simulink model "DynJointVerify"  (Simulink 7.6)
settings: Solver=ode45  StartTime=0.0  StopTime=8  RelTol=1e-3
InitFcn:
  | eval('Config.m')
values from neighbouring files (symbols this model uses):
  a2 = 0    [Config.m]    (also in CtrPlatformCfg.m)
  a3 = 0    [Config.m]    (also in CtrPlatformCfg.m)
  a4 = 0    [Config.m]    (also in CtrPlatformCfg.m)
  a5 = 90    [Config.m]    (also in CtrPlatformCfg.m)
  a6 = 0    [Config.m]    (also in CtrPlatformCfg.m)
  Cen = Cen(:)'    [Config.m]    (also in CtrPlatformCfg.m; DynEulerTest.m = Cen'; EfDynCAD.m = [cen1,cen2,cen3,cen4,cen5,cen6]')
  freq = tvel/radius    (= 1)    [Config.m]    (also in CtrPlatformCfg.m)
  Gravity = 9.8    [Config.m]    (also in CtrPlatformCfg.m)
  Ie1 = in1(:)'    [Config.m]    (also in CtrPlatformCfg.m; DynEulerTest.m = in1(:); EfDynCAD.m = in1(:))
  Ie2 = in2(:)'    [Config.m]    (also in CtrPlatformCfg.m; DynEulerTest.m = in2(:); EfDynCAD.m = in2(:))
  Ie3 = in3(:)'    [Config.m]    (also in CtrPlatformCfg.m; DynEulerTest.m = in3(:); EfDynCAD.m = in3(:))
  Ie4 = in4(:)'    [Config.m]    (also in CtrPlatformCfg.m; DynEulerTest.m = in4(:); EfDynCAD.m = in4(:))
  Ie5 = in5(:)'    [Config.m]    (also in CtrPlatformCfg.m; DynEulerTest.m = in5(:); EfDynCAD.m = in5(:))
  Ie6 = in6(:)'    [Config.m]    (also in CtrPlatformCfg.m; DynEulerTest.m = in6(:); EfDynCAD.m = in6(:))
  in1 = [5.2954 -0.2565 -0.6366;-0.2565 4.7000 0.2830;-0.6366 0.2829 5.8635]    [Config.m]    (also in CtrPlatformCfg.m; DynEulerTest.m; EfDynCAD.m = [0.54  -0.01 0.23)
  in2 = [5.8840 0.0072 0.0135;0.0072 6.0178 -0.1907;0.0135 -0.1907 0.3374]    [Config.m]    (also in CtrPlatformCfg.m; DynEulerTest.m; EfDynCAD.m = (R_x*R_z)*in2*(R_x*R_z)')
  in3 = [1.8201 -0.2274 -0.3112;-0.2274 2.2537 -0.1441;-0.3112 -0.1441 1.9485]    [Config.m]    (also in CtrPlatformCfg.m; DynEulerTest.m; EfDynCAD.m = (R_x*R_z)*in3*(R_x*R_z)')
  in4 = [0.0607 -0.0922 0;-0.0922 1.4493 0;0 0 1.4620]    [Config.m]    (also in CtrPlatformCfg.m; DynEulerTest.m = [0.0607 -0.0922 0;-0.0922 1.4493 0;0 0,1.4620]; EfDynCAD.m = (R_y*Rz)*in4*(R_y*Rz)')
  in5 = [0.0191 0.0032 0;0.0032 0.0228 0;0 0 0.0291]    [Config.m]    (also in CtrPlatformCfg.m; DynEulerTest.m; EfDynCAD.m = (R_x*R_y)*in5*(R_x*R_y)')
  in6 = [0.0012 0 0;0 0.0007 0;0 0 0.0007]    [Config.m]    (also in CtrPlatformCfg.m; DynEulerTest.m; EfDynCAD.m = (R_y*Rz)*in6*(R_y*Rz)')
  init_Endx = gd_init(1,4)    [Config.m]    (also in CtrPlatformCfg.m)
  init_Endy = gd_init(2,4)    [Config.m]    (also in CtrPlatformCfg.m)
  init_Endz = gd_init(3,4)    [Config.m]    (also in CtrPlatformCfg.m)
  init_Rot = gd_init(1:3,1:3)    [Config.m]    (also in CtrPlatformCfg.m)
  L = [l1 l2 l3 l4 l5 l6 l7 l8 l9]    [Config.m]    (also in CtrPlatformCfg.m)
  Ma = [ma1 ma2 ma3 ma4 ma5 ma6]    [Config.m]    (also in CtrPlatformCfg.m; DynEulerTest.m = [ma1; ma2; ma3; ma4; ma5; ma6]; EfDynCAD.m = [ma1 ma2 ma3 ma4 ma5 ma6]')
  tvel = 120    [Config.m]    (also in CtrPlatformCfg.m)
undefined symbols (not defined in the file or in its folder): a1, L_EU
libraries: mblibv1 x41, simulink x7
(part 2 of 2)

== system DynJointVerify/Dynamic/Largrange ==
  In1 : Inport
  BodyVel : Stateflow chart  TreatAsAtomicUnit=on
  C*Omega : Stateflow chart  TreatAsAtomicUnit=on
  Demux : Demux  Outputs=3
  M*Acc : Stateflow chart  TreatAsAtomicUnit=on
  N : Stateflow chart  TreatAsAtomicUnit=on
  Sum : Sum  Inputs=+++
  Force : Outport
  Acc : Outport  Port=2
  Potential : Outport  Port=3
  Cori : Outport  Port=4
  LaVel : Outport  Port=5
  wires:
  M*Acc/1(M_Acc) -> Sum/1, Acc/1
  C*Omega/1(C_Omega) -> Sum/3, Cori/1
  Demux/1 -> M*Acc/2(EnTheta), N/1(EnTheta), C*Omega/2(EnTheta), BodyVel/1(EnTheta)
  Demux/2 -> C*Omega/1(RefOmega), C*Omega/3(EnOmega), BodyVel/2(EnOmega)
  Demux/3 -> M*Acc/1(RefAcc)
  N/1(N) -> Sum/2, Potential/1
  In1/1 -> Demux/1
  Sum/1 -> Force/1
  BodyVel/1(Vel) -> LaVel/1

== system DynJointVerify/Dynamic/Potential Force ==
  In1 : Inport
  In2 : Inport  Port=2
  Demux : Demux  Outputs=6
  Demux1 : Demux  Outputs=6
  Err{1..6} (6 alike) : Scope
      Err1 settings: SaveName=ScopeData6
      Err2 settings: SaveName=ScopeData7
      Err3 settings: TimeRange=3  YMin=-6e-014  YMax=6e-014  SaveName=ScopeData8
      Err4 settings: SaveName=ScopeData9
      Err5 settings: SaveName=ScopeData10
      Err6 settings: SaveName=ScopeData11
  R1 Force : Scope  NumInputPorts=2
      settings: TimeRange=10  YMin=-2.999999999999999e-017~-1  YMax=4e-017~1
  R2 Force : Scope  NumInputPorts=2
      settings: YMin=-5~-5  YMax=5~5
  R3 Force : Scope  NumInputPorts=2
      settings: TimeRange=3  YMin=-227.5~-226.42678523  YMax=-225~-226.42678517  SaveName=ScopeData2
  R4 Force : Scope  NumInputPorts=2
      settings: YMin=-5~-5  YMax=5~5  SaveName=ScopeData3
  R5 Force : Scope  NumInputPorts=2
      settings: YMin=-5~-5  YMax=5~5  SaveName=ScopeData4
  R6 Force : Scope  NumInputPorts=2
      settings: YMin=-5~-5  YMax=5~5  SaveName=ScopeData5
  Sum{,1..5} (6 alike) : Sum  Inputs=+|-
  wires:
  In2/1 -> Demux1/1
  In1/1 -> Demux/1
  Sum/1 -> Err1/1
  Sum1/1 -> Err2/1
  Sum2/1 -> Err3/1
  Sum3/1 -> Err4/1
  Sum4/1 -> Err5/1
  Sum5/1 -> Err6/1
  Demux/1 -> Sum/1, R1 Force/1
  Demux1/1 -> Sum/2, R1 Force/2
  Demux/2 -> R2 Force/1, Sum1/1
  Demux/3 -> R3 Force/1, Sum2/1
  Demux/4 -> R4 Force/1, Sum3/1
  Demux/5 -> R5 Force/1, Sum4/1
  Demux/6 -> R6 Force/1, Sum5/1
  Demux1/2 -> R2 Force/2, Sum1/2
  Demux1/3 -> R3 Force/2, Sum2/2
  Demux1/4 -> R4 Force/2, Sum3/2
  Demux1/5 -> R5 Force/2, Sum4/2
  Demux1/6 -> R6 Force/2, Sum5/2

== system DynJointVerify/Error Analysis/Euler ==
  In1 : Inport
  In2 : Inport  Port=2
  Demux : Demux  Outputs=6
  Demux1 : Demux  Outputs=6
  Err{1..6} (6 alike) : Scope
      Err1 settings: SaveName=ScopeData6
      Err2 settings: SaveName=ScopeData7
      Err3 settings: TimeRange=3  YMin=-6e-014  YMax=6e-014  SaveName=ScopeData8
      Err4 settings: SaveName=ScopeData9
      Err5 settings: SaveName=ScopeData10
      Err6 settings: SaveName=ScopeData11
  R1 Force : Scope  NumInputPorts=2
      settings: TimeRange=10  YMin=-2.999999999999999e-017~-1  YMax=4e-017~1
  R2 Force : Scope  NumInputPorts=2
      settings: YMin=-5~-5  YMax=5~5
  R3 Force : Scope  NumInputPorts=2
      settings: TimeRange=3  YMin=-227.5~-226.42678523  YMax=-225~-226.42678517  SaveName=ScopeData2
  R4 Force : Scope  NumInputPorts=2
      settings: YMin=-5~-5  YMax=5~5  SaveName=ScopeData3
  R5 Force : Scope  NumInputPorts=2
      settings: YMin=-5~-5  YMax=5~5  SaveName=ScopeData4
  R6 Force : Scope  NumInputPorts=2
      settings: YMin=-5~-5  YMax=5~5  SaveName=ScopeData5
  Sum{,1..5} (6 alike) : Sum  Inputs=+|-
  wires:
  In2/1 -> Demux1/1
  In1/1 -> Demux/1
  Sum/1 -> Err1/1
  Sum1/1 -> Err2/1
  Sum2/1 -> Err3/1
  Sum3/1 -> Err4/1
  Sum4/1 -> Err5/1
  Sum5/1 -> Err6/1
  Demux/1 -> R1 Force/1, Sum/1
  Demux1/1 -> R1 Force/2, Sum/2
  Demux/2 -> Sum1/1, R2 Force/1
  Demux/3 -> Sum2/1, R3 Force/1
  Demux/4 -> Sum3/1, R4 Force/1
  Demux/5 -> Sum4/1, R5 Force/1
  Demux/6 -> Sum5/1, R6 Force/1
  Demux1/2 -> Sum1/2, R2 Force/2
  Demux1/3 -> Sum2/2, R3 Force/2
  Demux1/4 -> Sum3/2, R4 Force/2
  Demux1/5 -> Sum4/2, R5 Force/2
  Demux1/6 -> Sum5/2, R6 Force/2

== system DynJointVerify/Error Analysis/Largrange ==
  In1 : Inport
  In2 : Inport  Port=2
  Demux : Demux  Outputs=6
  Demux1 : Demux  Outputs=6
  Err{1..6} (6 alike) : Scope
      Err1 settings: SaveName=ScopeData6
      Err2 settings: SaveName=ScopeData7
      Err3 settings: TimeRange=3  YMin=-6e-014  YMax=6e-014  SaveName=ScopeData8
      Err4 settings: SaveName=ScopeData9
      Err5 settings: SaveName=ScopeData10
      Err6 settings: SaveName=ScopeData11
  R1 Force : Scope  NumInputPorts=2
      settings: TimeRange=10  YMin=-2.999999999999999e-017~-1  YMax=4e-017~1
  R2 Force : Scope  NumInputPorts=2
      settings: YMin=-5~-5  YMax=5~5
  R3 Force : Scope  NumInputPorts=2
      settings: TimeRange=3  YMin=-227.5~-226.42678523  YMax=-225~-226.42678517  SaveName=ScopeData2
  R4 Force : Scope  NumInputPorts=2
      settings: YMin=-5~-5  YMax=5~5  SaveName=ScopeData3
  R5 Force : Scope  NumInputPorts=2
      settings: YMin=-5~-5  YMax=5~5  SaveName=ScopeData4
  R6 Force : Scope  NumInputPorts=2
      settings: YMin=-5~-5  YMax=5~5  SaveName=ScopeData5
  Sum{,1..5} (6 alike) : Sum  Inputs=+|-
  wires:
  Sum/1 -> Err1/1
  Sum1/1 -> Err2/1
  Sum2/1 -> Err3/1
  Sum3/1 -> Err4/1
  Sum4/1 -> Err5/1
  Sum5/1 -> Err6/1
  Demux/1 -> Sum/1, R1 Force/1
  Demux1/1 -> Sum/2, R1 Force/2
  Demux/2 -> R2 Force/1, Sum1/1
  Demux/3 -> R3 Force/1, Sum2/1
  Demux/4 -> R4 Force/1, Sum3/1
  Demux/5 -> R5 Force/1, Sum4/1
  Demux/6 -> R6 Force/1, Sum5/1
  Demux1/2 -> R2 Force/2, Sum1/2
  Demux1/3 -> R3 Force/2, Sum2/2
  Demux1/4 -> R4 Force/2, Sum3/2
  Demux1/5 -> R5 Force/2, Sum4/2
  Demux1/6 -> R6 Force/2, Sum5/2
  In1/1 -> Demux/1
  In2/1 -> Demux1/1

== system DynJointVerify/Error Analysis/VelDisplay ==
  In1 : Inport
  In4 : Inport  Port=2
  Demux3 : Demux  Outputs=6
  Demux4 : Demux  Outputs=6
  Jnt1 : Subsystem
  Jnt2 : Subsystem
  Jnt3 : Subsystem
  Jnt4 : Subsystem
  Jnt5 : Subsystem
  Jnt6 : Subsystem
  wires:
  In1/1 -> Demux4/1
  In4/1 -> Demux3/1
  Demux4/1 -> Jnt1/1(In1)
  Demux3/1 -> Jnt1/2(In2)
  Demux4/2 -> Jnt2/1(In1)
  Demux3/2 -> Jnt2/2(In2)
  Demux4/3 -> Jnt3/1(In1)
  Demux3/3 -> Jnt3/2(In2)
  Demux4/4 -> Jnt4/1(In1)
  Demux3/4 -> Jnt4/2(In2)
  Demux4/5 -> Jnt5/1(In1)
  Demux3/5 -> Jnt5/2(In2)
  Demux4/6 -> Jnt6/1(In1)
  Demux3/6 -> Jnt6/2(In2)

== system DynJointVerify/Fanuc/ BodySensor 1 ==
  Avx : Scope
      settings: TimeRange=3  YMin=-150  YMax=125  SaveName=ScopeData62
  Avy : Scope
      settings: TimeRange=3  YMin=-150  YMax=125  SaveName=ScopeData63
  Avz : Scope
      settings: TimeRange=3  YMin=-150  YMax=125  SaveName=ScopeData64
  Awx : Scope
      settings: TimeRange=3  YMin=-150  YMax=125  SaveName=ScopeData65
  Awy : Scope
      settings: TimeRange=3  YMin=-150  YMax=125  SaveName=ScopeData66
  Awz : Scope
      settings: TimeRange=3  YMin=-150  YMax=125  SaveName=ScopeData67
  "Body Sensor " : mblibv1/Sensors &  Actuators/Body Sensor  DialogController=MECH.DynMechDlgSource  SystemSampleTime=-1  UpdateFromCAD=off  PhysicalDomain=Mechanical  PortType=blob  Muxed=on  Pose=off  Angle=on  AngleUnits=deg  ArcVelocity=on  ArcVelocityUnits=deg/s  ArcAcceleration=on  ArcAccelerationUnits=deg/s^2  CoordPosition=off  CoordPositionUnits=mm  Velocity=on  VelocityUnits=mm/s  Acceleration=on  AccelerationUnits=mm/s^2  Quaternion=on  QuaternionDT=off  QuaternionDDT=off  QuaternionUnits=off  OutputVector=[1]  ActiveIO=on  Width=12  DialogClass=MechanicalSensorBlock  ReferenceFrame=Local (Body CS)
  Demux5 : Demux  Outputs=12
  Vx : Scope
      settings: TimeRange=3  YMin=-150  YMax=125  SaveName=ScopeData55
  Vy : Scope
      settings: TimeRange=3  YMin=-150  YMax=125  SaveName=ScopeData57
  Vz : Scope
      settings: TimeRange=3  YMin=-150  YMax=125  SaveName=ScopeData58
  wx : Scope
      settings: TimeRange=3  YMin=-150  YMax=125  SaveName=ScopeData59
  wy : Scope
      settings: TimeRange=3  YMin=-150  YMax=125  SaveName=ScopeData60
  wz : Scope
      settings: TimeRange=3  YMin=-150  YMax=125  SaveName=ScopeData61
  Conn1 : PMIOPort  Port=1  Side=Left
  Out : Outport
  wires:
  "Body Sensor "/1 -> Out/1, Demux5/1
  Demux5/1 -> Vx/1
  Demux5/2 -> Vy/1
  Demux5/3 -> Vz/1
  Demux5/4 -> wx/1
  Demux5/5 -> wy/1
  Demux5/6 -> wz/1
  Demux5/7 -> Avx/1
  Demux5/8 -> Avy/1
  Demux5/9 -> Avz/1
  Demux5/10 -> Awx/1
  Demux5/11 -> Awy/1
  Demux5/12 -> Awz/1
  connections:
  Conn1/RConn1 -- "Body Sensor "/LConn1

== system DynJointVerify/Fanuc/ BodySensor 2 ==
  Avx : Scope
      settings: TimeRange=3  YMin=-150  YMax=125  SaveName=ScopeData62
  Avy : Scope
      settings: TimeRange=3  YMin=-150  YMax=125  SaveName=ScopeData63
  Avz : Scope
      settings: TimeRange=3  YMin=-150  YMax=125  SaveName=ScopeData64
  Awx : Scope
      settings: TimeRange=3  YMin=-150  YMax=125  SaveName=ScopeData65
  Awy : Scope
      settings: TimeRange=3  YMin=-150  YMax=125  SaveName=ScopeData66
  Awz : Scope
      settings: TimeRange=3  YMin=-150  YMax=125  SaveName=ScopeData67
  "Body Sensor " : mblibv1/Sensors &  Actuators/Body Sensor  DialogController=MECH.DynMechDlgSource  SystemSampleTime=-1  UpdateFromCAD=off  PhysicalDomain=Mechanical  PortType=blob  Muxed=on  Pose=off  Angle=on  AngleUnits=deg  ArcVelocity=on  ArcVelocityUnits=deg/s  ArcAcceleration=on  ArcAccelerationUnits=deg/s^2  CoordPosition=off  CoordPositionUnits=mm  Velocity=on  VelocityUnits=mm/s  Acceleration=on  AccelerationUnits=mm/s^2  Quaternion=on  QuaternionDT=off  QuaternionDDT=off  QuaternionUnits=off  OutputVector=[1]  ActiveIO=on  Width=12  DialogClass=MechanicalSensorBlock  ReferenceFrame=Local (Body CS)
  Demux5 : Demux  Outputs=12
  Vx : Scope
      settings: TimeRange=3  YMin=-150  YMax=125  SaveName=ScopeData55
  Vy : Scope
      settings: TimeRange=3  YMin=-150  YMax=125  SaveName=ScopeData57
  Vz : Scope
      settings: TimeRange=3  YMin=-150  YMax=125  SaveName=ScopeData58
  wx : Scope
      settings: TimeRange=3  YMin=-150  YMax=125  SaveName=ScopeData59
  wy : Scope
      settings: TimeRange=3  YMin=-150  YMax=125  SaveName=ScopeData60
  wz : Scope
      settings: TimeRange=3  YMin=-150  YMax=125  SaveName=ScopeData61
  Conn1 : PMIOPort  Port=1  Side=Left
  Out : Outport
  wires:
  Demux5/12 -> Awz/1
  Demux5/11 -> Awy/1
  Demux5/10 -> Awx/1
  Demux5/9 -> Avz/1
  Demux5/8 -> Avy/1
  Demux5/7 -> Avx/1
  Demux5/6 -> wz/1
  Demux5/5 -> wy/1
  Demux5/4 -> wx/1
  Demux5/3 -> Vz/1
  Demux5/2 -> Vy/1
  Demux5/1 -> Vx/1
  "Body Sensor "/1 -> Demux5/1, Out/1
  connections:
  Conn1/RConn1 -- "Body Sensor "/LConn1

== system DynJointVerify/Fanuc/ BodySensor 3 ==
  Avx : Scope
      settings: TimeRange=3  YMin=-150  YMax=125  SaveName=ScopeData62
  Avy : Scope
      settings: TimeRange=3  YMin=-150  YMax=125  SaveName=ScopeData63
  Avz : Scope
      settings: TimeRange=3  YMin=-150  YMax=125  SaveName=ScopeData64
  Awx : Scope
      settings: TimeRange=3  YMin=-150  YMax=125  SaveName=ScopeData65
  Awy : Scope
      settings: TimeRange=3  YMin=-150  YMax=125  SaveName=ScopeData66
  Awz : Scope
      settings: TimeRange=3  YMin=-150  YMax=125  SaveName=ScopeData67
  "Body Sensor " : mblibv1/Sensors &  Actuators/Body Sensor  DialogController=MECH.DynMechDlgSource  SystemSampleTime=-1  UpdateFromCAD=off  PhysicalDomain=Mechanical  PortType=blob  Muxed=on  Pose=off  Angle=on  AngleUnits=deg  ArcVelocity=on  ArcVelocityUnits=deg/s  ArcAcceleration=on  ArcAccelerationUnits=deg/s^2  CoordPosition=off  CoordPositionUnits=mm  Velocity=on  VelocityUnits=mm/s  Acceleration=on  AccelerationUnits=mm/s^2  Quaternion=on  QuaternionDT=off  QuaternionDDT=off  QuaternionUnits=off  OutputVector=[1]  ActiveIO=on  Width=12  DialogClass=MechanicalSensorBlock  ReferenceFrame=Local (Body CS)
  Demux5 : Demux  Outputs=12
  Vx : Scope
      settings: TimeRange=3  YMin=-150  YMax=125  SaveName=ScopeData55
  Vy : Scope
      settings: TimeRange=3  YMin=-150  YMax=125  SaveName=ScopeData57
  Vz : Scope
      settings: TimeRange=3  YMin=-150  YMax=125  SaveName=ScopeData58
  wx : Scope
      settings: TimeRange=3  YMin=-150  YMax=125  SaveName=ScopeData59
  wy : Scope
      settings: TimeRange=3  YMin=-150  YMax=125  SaveName=ScopeData60
  wz : Scope
      settings: TimeRange=3  YMin=-150  YMax=125  SaveName=ScopeData61
  Conn1 : PMIOPort  Port=1  Side=Left
  Out : Outport
  wires:
  "Body Sensor "/1 -> Out/1, Demux5/1
  Demux5/1 -> Vx/1
  Demux5/2 -> Vy/1
  Demux5/3 -> Vz/1
  Demux5/4 -> wx/1
  Demux5/5 -> wy/1
  Demux5/6 -> wz/1
  Demux5/7 -> Avx/1
  Demux5/8 -> Avy/1
  Demux5/9 -> Avz/1
  Demux5/10 -> Awx/1
  Demux5/11 -> Awy/1
  Demux5/12 -> Awz/1
  connections:
  Conn1/RConn1 -- "Body Sensor "/LConn1

== system DynJointVerify/Fanuc/ BodySensor 4 ==
  Avx : Scope
      settings: TimeRange=3  YMin=-150  YMax=125  SaveName=ScopeData62
  Avy : Scope
      settings: TimeRange=3  YMin=-150  YMax=125  SaveName=ScopeData63
  Avz : Scope
      settings: TimeRange=3  YMin=-150  YMax=125  SaveName=ScopeData64
  Awx : Scope
      settings: TimeRange=3  YMin=-150  YMax=125  SaveName=ScopeData65
  Awy : Scope
      settings: TimeRange=3  YMin=-150  YMax=125  SaveName=ScopeData66
  Awz : Scope
      settings: TimeRange=3  YMin=-150  YMax=125  SaveName=ScopeData67
  "Body Sensor " : mblibv1/Sensors &  Actuators/Body Sensor  DialogController=MECH.DynMechDlgSource  SystemSampleTime=-1  UpdateFromCAD=off  PhysicalDomain=Mechanical  PortType=blob  Muxed=on  Pose=off  Angle=on  AngleUnits=deg  ArcVelocity=on  ArcVelocityUnits=deg/s  ArcAcceleration=on  ArcAccelerationUnits=deg/s^2  CoordPosition=off  CoordPositionUnits=mm  Velocity=on  VelocityUnits=mm/s  Acceleration=on  AccelerationUnits=mm/s^2  Quaternion=on  QuaternionDT=off  QuaternionDDT=off  QuaternionUnits=off  OutputVector=[1]  ActiveIO=on  Width=12  DialogClass=MechanicalSensorBlock  ReferenceFrame=Local (Body CS)
  Demux5 : Demux  Outputs=12
  Vx : Scope
      settings: TimeRange=3  YMin=-150  YMax=125  SaveName=ScopeData55
  Vy : Scope
      settings: TimeRange=3  YMin=-150  YMax=125  SaveName=ScopeData57
  Vz : Scope
      settings: TimeRange=3  YMin=-150  YMax=125  SaveName=ScopeData58
  wx : Scope
      settings: TimeRange=3  YMin=-150  YMax=125  SaveName=ScopeData59
  wy : Scope
      settings: TimeRange=3  YMin=-150  YMax=125  SaveName=ScopeData60
  wz : Scope
      settings: TimeRange=3  YMin=-150  YMax=125  SaveName=ScopeData61
  Conn1 : PMIOPort  Port=1  Side=Left
  Out : Outport
  wires:
  Demux5/12 -> Awz/1
  Demux5/11 -> Awy/1
  Demux5/10 -> Awx/1
  Demux5/9 -> Avz/1
  Demux5/8 -> Avy/1
  Demux5/7 -> Avx/1
  Demux5/6 -> wz/1
  Demux5/5 -> wy/1
  Demux5/4 -> wx/1
  Demux5/3 -> Vz/1
  Demux5/2 -> Vy/1
  Demux5/1 -> Vx/1
  "Body Sensor "/1 -> Demux5/1, Out/1
  connections:
  Conn1/RConn1 -- "Body Sensor "/LConn1

== system DynJointVerify/Fanuc/ BodySensor 5 ==
  Avx : Scope
      settings: TimeRange=3  YMin=-150  YMax=125  SaveName=ScopeData62
  Avy : Scope
      settings: TimeRange=3  YMin=-150  YMax=125  SaveName=ScopeData63
  Avz : Scope
      settings: TimeRange=3  YMin=-150  YMax=125  SaveName=ScopeData64
  Awx : Scope
      settings: TimeRange=3  YMin=-150  YMax=125  SaveName=ScopeData65
  Awy : Scope
      settings: TimeRange=3  YMin=-150  YMax=125  SaveName=ScopeData66
  Awz : Scope
      settings: TimeRange=3  YMin=-150  YMax=125  SaveName=ScopeData67
  "Body Sensor " : mblibv1/Sensors &  Actuators/Body Sensor  DialogController=MECH.DynMechDlgSource  SystemSampleTime=-1  UpdateFromCAD=off  PhysicalDomain=Mechanical  PortType=blob  Muxed=on  Pose=off  Angle=on  AngleUnits=deg  ArcVelocity=on  ArcVelocityUnits=deg/s  ArcAcceleration=on  ArcAccelerationUnits=deg/s^2  CoordPosition=off  CoordPositionUnits=mm  Velocity=on  VelocityUnits=mm/s  Acceleration=on  AccelerationUnits=mm/s^2  Quaternion=on  QuaternionDT=off  QuaternionDDT=off  QuaternionUnits=off  OutputVector=[1]  ActiveIO=on  Width=12  DialogClass=MechanicalSensorBlock  ReferenceFrame=Local (Body CS)
  Demux5 : Demux  Outputs=12
  Vx : Scope
      settings: TimeRange=3  YMin=-150  YMax=125  SaveName=ScopeData55
  Vy : Scope
      settings: TimeRange=3  YMin=-150  YMax=125  SaveName=ScopeData57
  Vz : Scope
      settings: TimeRange=3  YMin=-150  YMax=125  SaveName=ScopeData58
  wx : Scope
      settings: TimeRange=3  YMin=-150  YMax=125  SaveName=ScopeData59
  wy : Scope
      settings: TimeRange=3  YMin=-150  YMax=125  SaveName=ScopeData60
  wz : Scope
      settings: TimeRange=3  YMin=-150  YMax=125  SaveName=ScopeData61
  Conn1 : PMIOPort  Port=1  Side=Left
  Out : Outport
  wires:
  "Body Sensor "/1 -> Out/1, Demux5/1
  Demux5/1 -> Vx/1
  Demux5/2 -> Vy/1
  Demux5/3 -> Vz/1
  Demux5/4 -> wx/1
  Demux5/5 -> wy/1
  Demux5/6 -> wz/1
  Demux5/7 -> Avx/1
  Demux5/8 -> Avy/1
  Demux5/9 -> Avz/1
  Demux5/10 -> Awx/1
  Demux5/11 -> Awy/1
  Demux5/12 -> Awz/1
  connections:
  Conn1/RConn1 -- "Body Sensor "/LConn1

== system DynJointVerify/Fanuc/ BodySensor 6 ==
  Avx : Scope
      settings: TimeRange=3  YMin=-150  YMax=125  SaveName=ScopeData62
  Avy : Scope
      settings: TimeRange=3  YMin=-150  YMax=125  SaveName=ScopeData63
  Avz : Scope
      settings: TimeRange=3  YMin=-150  YMax=125  SaveName=ScopeData64
  Awx : Scope
      settings: TimeRange=3  YMin=-150  YMax=125  SaveName=ScopeData65
  Awy : Scope
      settings: TimeRange=3  YMin=-150  YMax=125  SaveName=ScopeData66
  Awz : Scope
      settings: TimeRange=3  YMin=-150  YMax=125  SaveName=ScopeData67
  "Body Sensor " : mblibv1/Sensors &  Actuators/Body Sensor  DialogController=MECH.DynMechDlgSource  SystemSampleTime=-1  UpdateFromCAD=off  PhysicalDomain=Mechanical  PortType=blob  Muxed=on  Pose=off  Angle=on  AngleUnits=deg  ArcVelocity=on  ArcVelocityUnits=deg/s  ArcAcceleration=on  ArcAccelerationUnits=deg/s^2  CoordPosition=off  CoordPositionUnits=mm  Velocity=on  VelocityUnits=mm/s  Acceleration=on  AccelerationUnits=mm/s^2  Quaternion=on  QuaternionDT=off  QuaternionDDT=off  QuaternionUnits=off  OutputVector=[1]  ActiveIO=on  Width=12  DialogClass=MechanicalSensorBlock  ReferenceFrame=Local (Body CS)
  Demux5 : Demux  Outputs=12
  Vx : Scope
      settings: TimeRange=3  YMin=-150  YMax=125  SaveName=ScopeData55
  Vy : Scope
      settings: TimeRange=3  YMin=-150  YMax=125  SaveName=ScopeData57
  Vz : Scope
      settings: TimeRange=3  YMin=-150  YMax=125  SaveName=ScopeData58
  wx : Scope
      settings: TimeRange=3  YMin=-150  YMax=125  SaveName=ScopeData59
  wy : Scope
      settings: TimeRange=3  YMin=-150  YMax=125  SaveName=ScopeData60
  wz : Scope
      settings: TimeRange=3  YMin=-150  YMax=125  SaveName=ScopeData61
  Conn1 : PMIOPort  Port=1  Side=Left
  Out : Outport
  wires:
  Demux5/12 -> Awz/1
  Demux5/11 -> Awy/1
  Demux5/10 -> Awx/1
  Demux5/9 -> Avz/1
  Demux5/8 -> Avy/1
  Demux5/7 -> Avx/1
  Demux5/6 -> wz/1
  Demux5/5 -> wy/1
  Demux5/4 -> wx/1
  Demux5/3 -> Vz/1
  Demux5/2 -> Vy/1
  Demux5/1 -> Vx/1
  "Body Sensor "/1 -> Demux5/1, Out/1
  connections:
  Conn1/RConn1 -- "Body Sensor "/LConn1

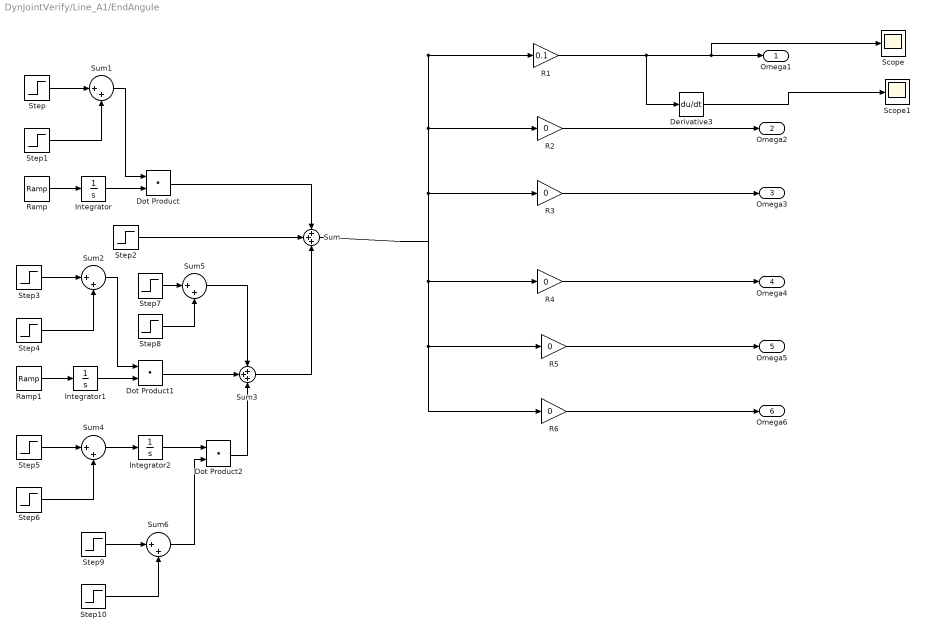
== system DynJointVerify/Line_A1/EndAngule ==
  Derivative3 : Derivative
  Dot Product : DotProduct  InputSameDT=on  OutDataTypeStr=Inherit: Inherit via internal rule
  Dot Product1 : DotProduct  InputSameDT=on  OutDataTypeStr=Inherit: Inherit via internal rule
  Dot Product2 : DotProduct  InputSameDT=on  OutDataTypeStr=Inherit: Inherit via internal rule
  Integrator : Integrator
  Integrator1 : Integrator
  Integrator2 : Integrator
  R1 : Gain  Gain=0.1
  R{2..6} (5 alike) : Gain  Gain=0
  Ramp : simulink/Sources/Ramp  SystemSampleTime=-1  slope=1  start=0  X0=0
  Ramp1 : simulink/Sources/Ramp  SystemSampleTime=-1  slope=-1  start=0  X0=0
  Scope : Scope
      settings: SaveName=ScopeData42
  Scope1 : Scope
      settings: SaveName=ScopeData43
  Step : Step  After=-1  SampleTime=0
  Step1 : Step  Time=0  SampleTime=0
  Step10 : Step  SampleTime=0
  Step2 : Step  Time=2  SampleTime=0
  Step3 : Step  Time=2  After=-1  SampleTime=0
  Step4 : Step  SampleTime=0
  Step5 : Step  Time=2  After=-2  SampleTime=0
  Step6 : Step  After=2  SampleTime=0
  Step7 : Step  Time=2  After=-1  SampleTime=0
  Step8 : Step  SampleTime=0
  Step9 : Step  Time=2  After=-1  SampleTime=0
  Sum : Sum  Inputs=+++
  Sum{1..2,4..6} (5 alike) : Sum  Inputs=|++
  Sum3 : Sum  Inputs=+++
  Omega1 : Outport
  Omega2 : Outport  Port=2
  Omega3 : Outport  Port=3
  Omega4 : Outport  Port=4
  Omega5 : Outport  Port=5
  Omega6 : Outport  Port=6
  wires:
  R4/1 -> Omega4/1
  R6/1 -> Omega6/1
  R5/1 -> Omega5/1
  R3/1 -> Omega3/1
  R2/1 -> Omega2/1
  Ramp/1 -> Integrator/1
  R1/1 -> Omega1/1, Scope/1, Derivative3/1
  Sum/1 -> R1/1, R2/1, R3/1, R4/1, R5/1, R6/1
  Integrator/1 -> Dot Product/2
  Step/1 -> Sum1/1
  Sum1/1 -> Dot Product/1
  Step1/1 -> Sum1/2
  Dot Product/1 -> Sum/1
  Step2/1 -> Sum/2
  Ramp1/1 -> Integrator1/1
  Integrator1/1 -> Dot Product1/2
  Step3/1 -> Sum2/1
  Sum2/1 -> Dot Product1/1
  Step4/1 -> Sum2/2
  Sum3/1 -> Sum/3
  Step5/1 -> Sum4/1
  Step6/1 -> Sum4/2
  Sum4/1 -> Integrator2/1
  Dot Product1/1 -> Sum3/2
  Step7/1 -> Sum5/1
  Step8/1 -> Sum5/2
  Sum5/1 -> Sum3/1
  Step9/1 -> Sum6/1
  Step10/1 -> Sum6/2
  Integrator2/1 -> Dot Product2/1
  Sum6/1 -> Dot Product2/2
  Dot Product2/1 -> Sum3/3
  Derivative3/1 -> Scope1/1

== system DynJointVerify/Line_A23/EndAngule ==
  Dot Product : DotProduct  InputSameDT=on  OutDataTypeStr=Inherit: Inherit via internal rule
  Integrator : Integrator
  R{1..2,4..6} (5 alike) : Gain  Gain=0
  R3 : Gain  Gain=0.1
  Ramp : simulink/Sources/Ramp  SystemSampleTime=-1  slope=1  start=0  X0=0
  Step : Step  After=-2  SampleTime=0
  Step1 : Step  Time=0  After=2  SampleTime=0
  Step2 : Step  SampleTime=0
  Sum : Sum  Inputs=|++
  Sum1 : Sum  Inputs=|++
  Omega1 : Outport
  Omega2 : Outport  Port=2
  Omega3 : Outport  Port=3
  Omega4 : Outport  Port=4
  Omega5 : Outport  Port=5
  Omega6 : Outport  Port=6
  wires:
  Step1/1 -> Sum1/2
  Step2/1 -> Sum/2
  Dot Product/1 -> Sum/1
  Sum1/1 -> Dot Product/1
  Step/1 -> Sum1/1
  Integrator/1 -> Dot Product/2
  Sum/1 -> R6/1, R5/1, R4/1, R3/1, R2/1, R1/1
  R1/1 -> Omega1/1
  Ramp/1 -> Integrator/1
  R2/1 -> Omega2/1
  R3/1 -> Omega3/1
  R5/1 -> Omega5/1
  R6/1 -> Omega6/1
  R4/1 -> Omega4/1

== system DynJointVerify/Line_XZ/EndVelocity ==
  End_Vx : Constant  Value=30
  End_Vy : Constant  Value=0
  End_Vz : Constant  Value=-30
  EndVx : Outport
  EndVy : Outport  Port=2
  EndVz : Outport  Port=3
  wires:
  End_Vy/1 -> EndVy/1
  End_Vz/1 -> EndVz/1
  End_Vx/1 -> EndVx/1

== system DynJointVerify/Still/EndVelocity ==
  Constant : Constant  Value=0
  Constant1 : Constant  Value=0
  Constant2 : Constant  Value=0
  EndVx : Outport
  EndVy : Outport  Port=2
  EndVz : Outport  Port=3
  wires:
  Constant/1 -> EndVx/1
  Constant1/1 -> EndVy/1
  Constant2/1 -> EndVz/1

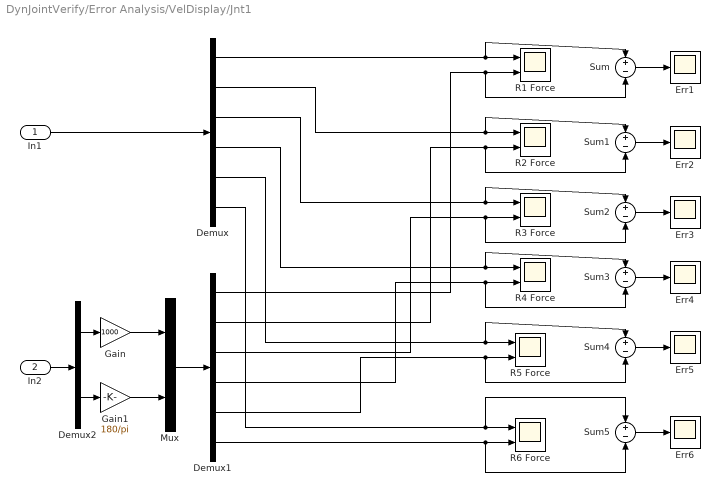
== system DynJointVerify/Error Analysis/VelDisplay/Jnt1 ==
  In1 : Inport
  In2 : Inport  Port=2
  Demux : Demux  Outputs=6
  Demux1 : Demux  Outputs=6
  Demux2 : Demux  Outputs=2
  Err{1..6} (6 alike) : Scope
      Err1 settings: SaveName=ScopeData6
      Err2 settings: SaveName=ScopeData7
      Err3 settings: TimeRange=3  YMin=-6e-014  YMax=6e-014  SaveName=ScopeData8
      Err4 settings: SaveName=ScopeData9
      Err5 settings: SaveName=ScopeData10
      Err6 settings: SaveName=ScopeData11
  Gain : Gain  Gain=1000
  Gain1 : Gain  Gain=180/pi
  Mux : Mux  Inputs=2
  R1 Force : Scope  NumInputPorts=2
      settings: TimeRange=3  YMin=-1400~-1000  YMax=600~400
  R2 Force : Scope  NumInputPorts=2
      settings: YMin=-5~-5  YMax=5~5
  R3 Force : Scope  NumInputPorts=2
      settings: TimeRange=3  YMin=-227.5~-226.42678523  YMax=-225~-226.42678517  SaveName=ScopeData2
  R4 Force : Scope  NumInputPorts=2
      settings: YMin=-5~-5  YMax=5~5  SaveName=ScopeData3
  R5 Force : Scope  NumInputPorts=2
      settings: YMin=-5~-5  YMax=5~5  SaveName=ScopeData4
  R6 Force : Scope  NumInputPorts=2
      settings: YMin=-5~-5  YMax=5~5  SaveName=ScopeData5
  Sum{,1..5} (6 alike) : Sum  Inputs=+|-
  wires:
  In1/1 -> Demux/1
  Sum/1 -> Err1/1
  Sum1/1 -> Err2/1
  Sum2/1 -> Err3/1
  Sum3/1 -> Err4/1
  Sum4/1 -> Err5/1
  Sum5/1 -> Err6/1
  Demux/1 -> Sum/1, R1 Force/1
  Demux1/1 -> Sum/2, R1 Force/2
  Demux/2 -> R2 Force/1, Sum1/1
  Demux/3 -> R3 Force/1, Sum2/1
  Demux/4 -> R4 Force/1, Sum3/1
  Demux/5 -> R5 Force/1, Sum4/1
  Demux/6 -> R6 Force/1, Sum5/1
  Demux1/2 -> R2 Force/2, Sum1/2
  Demux1/3 -> R3 Force/2, Sum2/2
  Demux1/4 -> R4 Force/2, Sum3/2
  Demux1/5 -> R5 Force/2, Sum4/2
  Demux1/6 -> R6 Force/2, Sum5/2
  Demux2/1 -> Gain/1
  Demux2/2 -> Gain1/1
  Gain/1 -> Mux/1
  Gain1/1 -> Mux/2
  In2/1 -> Demux2/1
  Mux/1 -> Demux1/1

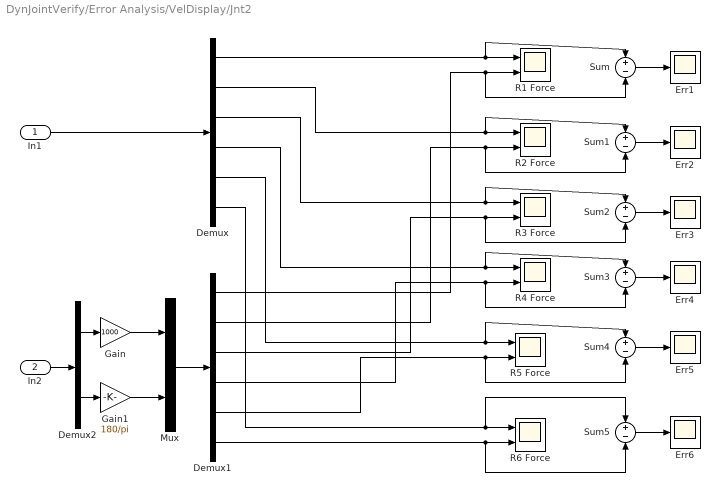
== system DynJointVerify/Error Analysis/VelDisplay/Jnt2 ==
  In1 : Inport
  In2 : Inport  Port=2
  Demux : Demux  Outputs=6
  Demux1 : Demux  Outputs=6
  Demux2 : Demux  Outputs=2
  Err{1..6} (6 alike) : Scope
      Err1 settings: TimeRange=3  SaveName=ScopeData6
      Err2 settings: SaveName=ScopeData7
      Err3 settings: TimeRange=3  YMin=-6e-014  YMax=6e-014  SaveName=ScopeData8
      Err4 settings: SaveName=ScopeData9
      Err5 settings: SaveName=ScopeData10
      Err6 settings: SaveName=ScopeData11
  Gain : Gain  Gain=1000
  Gain1 : Gain  Gain=180/pi
  Mux : Mux  Inputs=2
  R1 Force : Scope  NumInputPorts=2
      settings: TimeRange=3  YMin=-1400~-1000  YMax=600~400
  R2 Force : Scope  NumInputPorts=2
      settings: YMin=-5~-5  YMax=5~5
  R3 Force : Scope  NumInputPorts=2
      settings: TimeRange=3  YMin=-227.5~-226.42678523  YMax=-225~-226.42678517  SaveName=ScopeData2
  R4 Force : Scope  NumInputPorts=2
      settings: YMin=-5~-5  YMax=5~5  SaveName=ScopeData3
  R5 Force : Scope  NumInputPorts=2
      settings: YMin=-5~-5  YMax=5~5  SaveName=ScopeData4
  R6 Force : Scope  NumInputPorts=2
      settings: YMin=-5~-5  YMax=5~5  SaveName=ScopeData5
  Sum{,1..5} (6 alike) : Sum  Inputs=+|-
  wires:
  Mux/1 -> Demux1/1
  In2/1 -> Demux2/1
  Gain1/1 -> Mux/2
  Gain/1 -> Mux/1
  Demux2/2 -> Gain1/1
  Demux2/1 -> Gain/1
  Demux1/6 -> Sum5/2, R6 Force/2
  Demux1/5 -> Sum4/2, R5 Force/2
  Demux1/4 -> Sum3/2, R4 Force/2
  Demux1/3 -> Sum2/2, R3 Force/2
  Demux1/2 -> Sum1/2, R2 Force/2
  Demux/6 -> Sum5/1, R6 Force/1
  Demux/5 -> Sum4/1, R5 Force/1
  Demux/4 -> Sum3/1, R4 Force/1
  Demux/3 -> Sum2/1, R3 Force/1
  Demux/2 -> Sum1/1, R2 Force/1
  Demux1/1 -> R1 Force/2, Sum/2
  Demux/1 -> R1 Force/1, Sum/1
  Sum5/1 -> Err6/1
  Sum4/1 -> Err5/1
  Sum3/1 -> Err4/1
  Sum2/1 -> Err3/1
  Sum1/1 -> Err2/1
  Sum/1 -> Err1/1
  In1/1 -> Demux/1

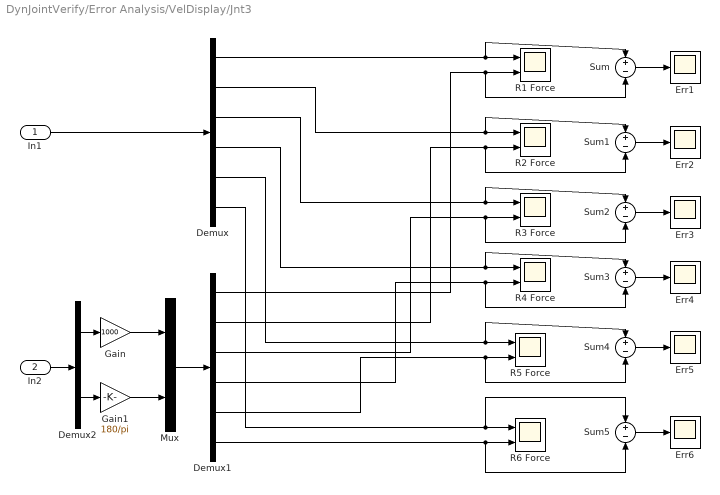
== system DynJointVerify/Error Analysis/VelDisplay/Jnt3 ==
  In1 : Inport
  In2 : Inport  Port=2
  Demux : Demux  Outputs=6
  Demux1 : Demux  Outputs=6
  Demux2 : Demux  Outputs=2
  Err{1..6} (6 alike) : Scope
      Err1 settings: SaveName=ScopeData6
      Err2 settings: SaveName=ScopeData7
      Err3 settings: TimeRange=3  YMin=-6e-014  YMax=6e-014  SaveName=ScopeData8
      Err4 settings: SaveName=ScopeData9
      Err5 settings: SaveName=ScopeData10
      Err6 settings: SaveName=ScopeData11
  Gain : Gain  Gain=1000
  Gain1 : Gain  Gain=180/pi
  Mux : Mux  Inputs=2
  R1 Force : Scope  NumInputPorts=2
      settings: TimeRange=3  YMin=-1400~-1000  YMax=600~400
  R2 Force : Scope  NumInputPorts=2
      settings: YMin=-5~-5  YMax=5~5
  R3 Force : Scope  NumInputPorts=2
      settings: TimeRange=3  YMin=-227.5~-226.42678523  YMax=-225~-226.42678517  SaveName=ScopeData2
  R4 Force : Scope  NumInputPorts=2
      settings: YMin=-5~-5  YMax=5~5  SaveName=ScopeData3
  R5 Force : Scope  NumInputPorts=2
      settings: YMin=-5~-5  YMax=5~5  SaveName=ScopeData4
  R6 Force : Scope  NumInputPorts=2
      settings: YMin=-5~-5  YMax=5~5  SaveName=ScopeData5
  Sum{,1..5} (6 alike) : Sum  Inputs=+|-
  wires:
  In1/1 -> Demux/1
  Sum/1 -> Err1/1
  Sum1/1 -> Err2/1
  Sum2/1 -> Err3/1
  Sum3/1 -> Err4/1
  Sum4/1 -> Err5/1
  Sum5/1 -> Err6/1
  Demux/1 -> Sum/1, R1 Force/1
  Demux1/1 -> Sum/2, R1 Force/2
  Demux/2 -> R2 Force/1, Sum1/1
  Demux/3 -> R3 Force/1, Sum2/1
  Demux/4 -> R4 Force/1, Sum3/1
  Demux/5 -> R5 Force/1, Sum4/1
  Demux/6 -> R6 Force/1, Sum5/1
  Demux1/2 -> R2 Force/2, Sum1/2
  Demux1/3 -> R3 Force/2, Sum2/2
  Demux1/4 -> R4 Force/2, Sum3/2
  Demux1/5 -> R5 Force/2, Sum4/2
  Demux1/6 -> R6 Force/2, Sum5/2
  Demux2/1 -> Gain/1
  Demux2/2 -> Gain1/1
  Gain/1 -> Mux/1
  Gain1/1 -> Mux/2
  In2/1 -> Demux2/1
  Mux/1 -> Demux1/1

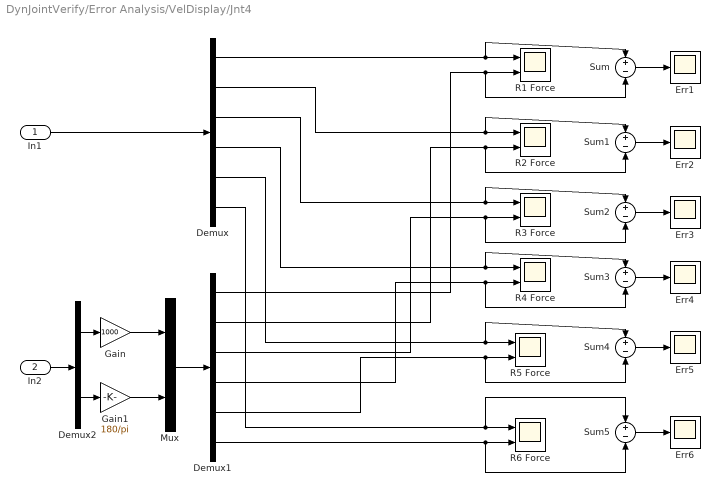
== system DynJointVerify/Error Analysis/VelDisplay/Jnt4 ==
  In1 : Inport
  In2 : Inport  Port=2
  Demux : Demux  Outputs=6
  Demux1 : Demux  Outputs=6
  Demux2 : Demux  Outputs=2
  Err{1..6} (6 alike) : Scope
      Err1 settings: SaveName=ScopeData6
      Err2 settings: SaveName=ScopeData7
      Err3 settings: TimeRange=3  YMin=-6e-014  YMax=6e-014  SaveName=ScopeData8
      Err4 settings: SaveName=ScopeData9
      Err5 settings: SaveName=ScopeData10
      Err6 settings: SaveName=ScopeData11
  Gain : Gain  Gain=1000
  Gain1 : Gain  Gain=180/pi
  Mux : Mux  Inputs=2
  R1 Force : Scope  NumInputPorts=2
      settings: TimeRange=3  YMin=-1400~-1000  YMax=600~400
  R2 Force : Scope  NumInputPorts=2
      settings: YMin=-5~-5  YMax=5~5
  R3 Force : Scope  NumInputPorts=2
      settings: TimeRange=3  YMin=-227.5~-226.42678523  YMax=-225~-226.42678517  SaveName=ScopeData2
  R4 Force : Scope  NumInputPorts=2
      settings: YMin=-5~-5  YMax=5~5  SaveName=ScopeData3
  R5 Force : Scope  NumInputPorts=2
      settings: YMin=-5~-5  YMax=5~5  SaveName=ScopeData4
  R6 Force : Scope  NumInputPorts=2
      settings: YMin=-5~-5  YMax=5~5  SaveName=ScopeData5
  Sum{,1..5} (6 alike) : Sum  Inputs=+|-
  wires:
  Mux/1 -> Demux1/1
  In2/1 -> Demux2/1
  Gain1/1 -> Mux/2
  Gain/1 -> Mux/1
  Demux2/2 -> Gain1/1
  Demux2/1 -> Gain/1
  Demux1/6 -> Sum5/2, R6 Force/2
  Demux1/5 -> Sum4/2, R5 Force/2
  Demux1/4 -> Sum3/2, R4 Force/2
  Demux1/3 -> Sum2/2, R3 Force/2
  Demux1/2 -> Sum1/2, R2 Force/2
  Demux/6 -> Sum5/1, R6 Force/1
  Demux/5 -> Sum4/1, R5 Force/1
  Demux/4 -> Sum3/1, R4 Force/1
  Demux/3 -> Sum2/1, R3 Force/1
  Demux/2 -> Sum1/1, R2 Force/1
  Demux1/1 -> R1 Force/2, Sum/2
  Demux/1 -> R1 Force/1, Sum/1
  Sum5/1 -> Err6/1
  Sum4/1 -> Err5/1
  Sum3/1 -> Err4/1
  Sum2/1 -> Err3/1
  Sum1/1 -> Err2/1
  Sum/1 -> Err1/1
  In1/1 -> Demux/1

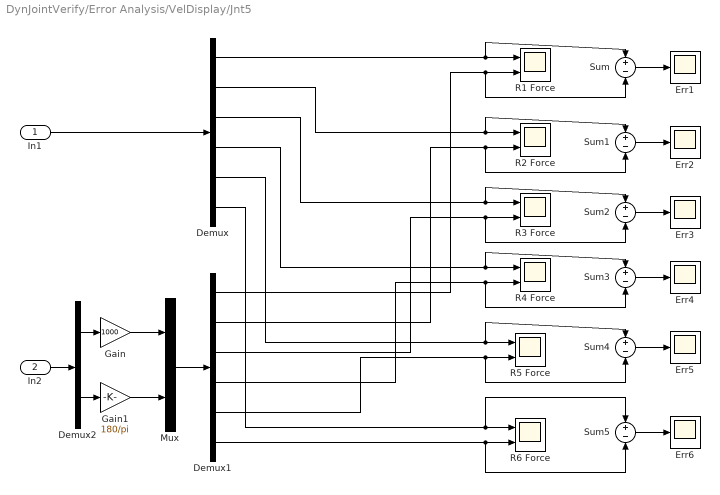
== system DynJointVerify/Error Analysis/VelDisplay/Jnt5 ==
  In1 : Inport
  In2 : Inport  Port=2
  Demux : Demux  Outputs=6
  Demux1 : Demux  Outputs=6
  Demux2 : Demux  Outputs=2
  Err{1..6} (6 alike) : Scope
      Err1 settings: SaveName=ScopeData6
      Err2 settings: SaveName=ScopeData7
      Err3 settings: TimeRange=3  YMin=-6e-014  YMax=6e-014  SaveName=ScopeData8
      Err4 settings: SaveName=ScopeData9
      Err5 settings: SaveName=ScopeData10
      Err6 settings: SaveName=ScopeData11
  Gain : Gain  Gain=1000
  Gain1 : Gain  Gain=180/pi
  Mux : Mux  Inputs=2
  R1 Force : Scope  NumInputPorts=2
      settings: TimeRange=3  YMin=-1400~-1000  YMax=600~400
  R2 Force : Scope  NumInputPorts=2
      settings: YMin=-5~-5  YMax=5~5
  R3 Force : Scope  NumInputPorts=2
      settings: TimeRange=3  YMin=-227.5~-226.42678523  YMax=-225~-226.42678517  SaveName=ScopeData2
  R4 Force : Scope  NumInputPorts=2
      settings: YMin=-5~-5  YMax=5~5  SaveName=ScopeData3
  R5 Force : Scope  NumInputPorts=2
      settings: YMin=-5~-5  YMax=5~5  SaveName=ScopeData4
  R6 Force : Scope  NumInputPorts=2
      settings: YMin=-5~-5  YMax=5~5  SaveName=ScopeData5
  Sum{,1..5} (6 alike) : Sum  Inputs=+|-
  wires:
  In1/1 -> Demux/1
  Sum/1 -> Err1/1
  Sum1/1 -> Err2/1
  Sum2/1 -> Err3/1
  Sum3/1 -> Err4/1
  Sum4/1 -> Err5/1
  Sum5/1 -> Err6/1
  Demux/1 -> Sum/1, R1 Force/1
  Demux1/1 -> Sum/2, R1 Force/2
  Demux/2 -> R2 Force/1, Sum1/1
  Demux/3 -> R3 Force/1, Sum2/1
  Demux/4 -> R4 Force/1, Sum3/1
  Demux/5 -> R5 Force/1, Sum4/1
  Demux/6 -> R6 Force/1, Sum5/1
  Demux1/2 -> R2 Force/2, Sum1/2
  Demux1/3 -> R3 Force/2, Sum2/2
  Demux1/4 -> R4 Force/2, Sum3/2
  Demux1/5 -> R5 Force/2, Sum4/2
  Demux1/6 -> R6 Force/2, Sum5/2
  Demux2/1 -> Gain/1
  Demux2/2 -> Gain1/1
  Gain/1 -> Mux/1
  Gain1/1 -> Mux/2
  In2/1 -> Demux2/1
  Mux/1 -> Demux1/1

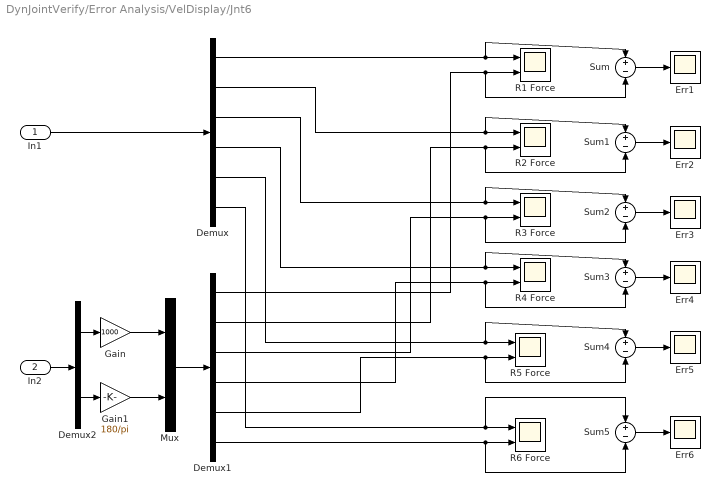
== system DynJointVerify/Error Analysis/VelDisplay/Jnt6 ==
  In1 : Inport
  In2 : Inport  Port=2
  Demux : Demux  Outputs=6
  Demux1 : Demux  Outputs=6
  Demux2 : Demux  Outputs=2
  Err{1..6} (6 alike) : Scope
      Err1 settings: SaveName=ScopeData6
      Err2 settings: SaveName=ScopeData7
      Err3 settings: TimeRange=3  YMin=-6e-014  YMax=6e-014  SaveName=ScopeData8
      Err4 settings: SaveName=ScopeData9
      Err5 settings: SaveName=ScopeData10
      Err6 settings: SaveName=ScopeData11
  Gain : Gain  Gain=1000
  Gain1 : Gain  Gain=180/pi
  Mux : Mux  Inputs=2
  R1 Force : Scope  NumInputPorts=2
      settings: TimeRange=3  YMin=-1400~-1000  YMax=600~400
  R2 Force : Scope  NumInputPorts=2
      settings: YMin=-5~-5  YMax=5~5
  R3 Force : Scope  NumInputPorts=2
      settings: TimeRange=3  YMin=-227.5~-226.42678523  YMax=-225~-226.42678517  SaveName=ScopeData2
  R4 Force : Scope  NumInputPorts=2
      settings: YMin=-5~-5  YMax=5~5  SaveName=ScopeData3
  R5 Force : Scope  NumInputPorts=2
      settings: YMin=-5~-5  YMax=5~5  SaveName=ScopeData4
  R6 Force : Scope  NumInputPorts=2
      settings: YMin=-5~-5  YMax=5~5  SaveName=ScopeData5
  Sum{,1..5} (6 alike) : Sum  Inputs=+|-
  wires:
  Mux/1 -> Demux1/1
  In2/1 -> Demux2/1
  Gain1/1 -> Mux/2
  Gain/1 -> Mux/1
  Demux2/2 -> Gain1/1
  Demux2/1 -> Gain/1
  Demux1/6 -> Sum5/2, R6 Force/2
  Demux1/5 -> Sum4/2, R5 Force/2
  Demux1/4 -> Sum3/2, R4 Force/2
  Demux1/3 -> Sum2/2, R3 Force/2
  Demux1/2 -> Sum1/2, R2 Force/2
  Demux/6 -> Sum5/1, R6 Force/1
  Demux/5 -> Sum4/1, R5 Force/1
  Demux/4 -> Sum3/1, R4 Force/1
  Demux/3 -> Sum2/1, R3 Force/1
  Demux/2 -> Sum1/1, R2 Force/1
  Demux1/1 -> R1 Force/2, Sum/2
  Demux/1 -> R1 Force/1, Sum/1
  Sum5/1 -> Err6/1
  Sum4/1 -> Err5/1
  Sum3/1 -> Err4/1
  Sum2/1 -> Err3/1
  Sum1/1 -> Err2/1
  Sum/1 -> Err1/1
  In1/1 -> Demux/1

== matlab function Circle_XY/Jacobian ==
  data: Omega output double; EndVel input double; Theta input double; L parameter double
function Omega = fcn(EndVel,Theta,L)
%#eml

Omega = zeros(6,1);
V = [EndVel; 0; 0; 0];   
g = fwd_kin(L,Theta');
Jb = body_Jacobian(L,Theta');
Adg_inv = double(AdjointInv(g));
Omega = double((Jb \ Adg_inv* V)')';

== matlab function Circle_XY/Inverse Kinematic ==
  data: EndPos input double; init_Rot parameter double; theta output double; L parameter double
function theta = fcn(EndPos,init_Rot,L)
%#eml
theta =[0;0; 0; 0; 0; 0];
gd = [init_Rot,EndPos;[0 0 0],1];
[theta_total,num_total] = inv_kin(gd,L);
theta = theta_total(:,2);

== matlab function Dynamic/Largrange/M*Acc ==
  data: RefAcc input double; EnTheta input double; M_Acc output double; L parameter double; Cen parameter double; Ma parameter double; Ie1 parameter double; Ie2 parameter double; Ie3 parameter double; Ie4 parameter double; Ie5 parameter double; Ie6 parameter double
function M_Acc = fcn(RefAcc,EnTheta,L,Cen,Ma,Ie1,Ie2,Ie3,Ie4,Ie5,Ie6)
%#eml

M_Acc = zeros(6,1);
M_Acc = M_d(L/1000,EnTheta',Cen,Ma,Ie1,Ie2,Ie3,Ie4,Ie5,Ie6)*RefAcc;

== matlab function Dynamic/Largrange/C*Omega ==
  data: RefOmega input double; C_Omega output double; EnTheta input double; EnOmega input double; L parameter double; Cen parameter double; Ma parameter double; Ie1 parameter double; Ie2 parameter double; Ie3 parameter double; Ie4 parameter double; Ie5 parameter double; Ie6 parameter double
function C_Omega = fcn(RefOmega,EnTheta,EnOmega,L,Cen,Ma,Ie1,Ie2,Ie3,Ie4,Ie5,Ie6)
%#eml

C_Omega =zeros(6,1);

L=L/1000;
M_dp = zeros(6,6*6);
M_dp(:,1:6) = M_dp1(L,EnTheta',Cen,Ma,Ie1,Ie2,Ie3,Ie4,Ie5,Ie6);
M_dp(:,7:12) = M_dp2(L,EnTheta',Cen,Ma,Ie1,Ie2,Ie3,Ie4,Ie5,Ie6);
M_dp(:,13:18) = M_dp3(L,EnTheta',Cen,Ma,Ie1,Ie2,Ie3,Ie4,Ie5,Ie6);
M_dp(:,19:24)= M_dp4(L,EnTheta',Cen,Ma,Ie1,Ie2,Ie3,Ie4,Ie5,Ie6);
M_dp(:,25:30) = M_dp5(L,EnTheta',Cen,Ma,Ie1,Ie2,Ie3,Ie4,Ie5,Ie6);
M_dp(:,31:36) = M_dp6(L,EnTheta',Cen,Ma,Ie1,Ie2,Ie3,Ie4,Ie5,Ie6);

C = zeros(6,6);

for i=1:6
    for j=1:6
        for k=1:6
                 C(i,j) =C(i,j)+ 0.5*(M_dp(i,(k-1)*6+j)+M_dp(i,(j-1)*6+k)-M_dp(k,(i-1)*6+j))*EnOmega(k);
            
        end
    end
end
C_Omega = C*RefOmega;
% end

== matlab function Dynamic/Largrange/N ==
  data: EnTheta input double; N output double; L parameter double; Cen parameter double; Ma parameter double; Gravity parameter double
function N = fcn(EnTheta,L,Cen,Ma,Gravity)
%#eml
N=zeros(6,1);
N=N_d(L/1000,EnTheta',Cen,Ma,Gravity);

== matlab function Line_A23/Forward ==
  data: Theta input double; EndPos output double; L parameter double
function EndPos = fcn(Theta,L)
%#eml
gd = fwd_kin(L,Theta');
EndPos = gd(1:3,4);

== matlab function Line_A23/Jacobian ==
  data: Theta input double; Omega input double; EndVel output double; L parameter double
function EndVel = fcn(Theta,Omega,L)
%#eml


EndVW = spat_Jacobian(L,Theta')*Omega;
gd = fwd_kin(L,Theta');
EndW = EndVW(4:6,1);
gd_pos = gd(1:3,4);
EndVel=cross(EndW,gd_pos);

== matlab function Line_XZ/Inverse Kinematic ==
  data: EndPos input double; init_Rot parameter double; theta output double; L parameter double
function theta = fcn(EndPos,init_Rot,L)
%#eml
theta =[0;0; 0; 0; 0; 0];
gd = [init_Rot,EndPos;[0 0 0],1];
[theta_total,num_total] = inv_kin(gd,L);
theta = theta_total(:,2);

== matlab function Line_XZ/Jacobian ==
  data: Omega output double; EndVel input double; Theta input double; L parameter double
function Omega = fcn(EndVel,Theta,L)
%#eml

Omega = zeros(6,1);
V = [EndVel; 0; 0; 0];   
g = fwd_kin(L,Theta');
Jb = body_Jacobian(L,Theta');
Adg_inv = double(AdjointInv(g));
Omega = double((Jb \ Adg_inv* V)')';

== matlab function Circle_YZ/Inverse Kinematic ==
  data: EndPos input double; init_Rot parameter double; theta output double; L parameter double
function theta = fcn(EndPos,init_Rot,L)
%#eml
theta =[0;0; 0; 0; 0; 0];
gd = [init_Rot,EndPos;[0 0 0],1];
[theta_total,num_total] = inv_kin(gd,L);
theta = theta_total(:,2);

== matlab function Circle_YZ/Jacobian ==
  data: Omega output double; EndVel input double; Theta input double; L parameter double
function Omega = fcn(EndVel,Theta,L)
%#eml

Omega = zeros(6,1);
V = [EndVel; 0; 0; 0];   
g = fwd_kin(L,Theta');
Jb = body_Jacobian(L,Theta');
Adg_inv = double(AdjointInv(g));
Omega = double((Jb \ Adg_inv* V)')';

== matlab function Line_A1/Forward ==
  data: Theta input double; EndPos output double; L parameter double
function EndPos = fcn(Theta,L)
%#eml
gd = fwd_kin(L,Theta');
EndPos = gd(1:3,4);

== matlab function Line_A1/Jacobian ==
  data: Theta input double; Omega input double; EndVel output double; L parameter double
function EndVel = fcn(Theta,Omega,L)
%#eml


EndVW = spat_Jacobian(L,Theta')*Omega;
gd = fwd_kin(L,Theta');
EndW = EndVW(4:6,1);
gd_pos = gd(1:3,4);
EndVel=cross(EndW,gd_pos);

== matlab function Still/Inverse Kinematic ==
  data: EndPos input double; init_Rot parameter double; theta output double; L parameter double
function theta = fcn(EndPos,init_Rot,L)
%#eml
theta =[0;0; 0; 0; 0; 0];
gd = [init_Rot,EndPos;[0 0 0],1];
[theta_total,num_total] = inv_kin(gd,L);
theta = theta_total(:,2);

== matlab function Still/Jacobian ==
  data: Omega output double; EndVel input double; Theta input double; L parameter double
function Omega = fcn(EndVel,Theta,L)
%#eml

Omega = zeros(6,1);
V = [EndVel; 0; 0; 0];   
g = fwd_kin(L,Theta');
Jb = body_Jacobian(L,Theta');
Adg_inv = double(AdjointInv(g));
Omega = double((Jb \ Adg_inv* V)')';

== matlab function Dynamic/Euler/C*Omega ==
  data: RefOmega input double; C_Omega output double; EnTheta input double; EnOmega input double; L_EU parameter double; Cen parameter double; Ma parameter double; Ie1 parameter double; Ie2 parameter double; Ie3 parameter double; Ie4 parameter double; Ie5 parameter double; Ie6 parameter double
function C_Omega = fcn(RefOmega,EnTheta,EnOmega,L_EU,Cen,Ma,Ie1,Ie2,Ie3,Ie4,Ie5,Ie6)
%#eml

C_Omega =zeros(6,1);

C_Omega = EulerCd(L_EU,Ma,Cen,Ie1,Ie2,Ie3,Ie4,Ie5,Ie6,EnTheta',EnOmega')*RefOmega;
% end

== matlab function Dynamic/Euler/M*Acc ==
  data: RefAcc input double; EnTheta input double; M_Acc output double; L_EU parameter double; Cen parameter double; Ma parameter double; Ie1 parameter double; Ie2 parameter double; Ie3 parameter double; Ie4 parameter double; Ie5 parameter double; Ie6 parameter double
function M_Acc = fcn(RefAcc,EnTheta,L_EU,Cen,Ma,Ie1,Ie2,Ie3,Ie4,Ie5,Ie6)
%#eml

M_Acc = zeros(6,1);
M_Acc = EulerMd(L_EU,Ma,Cen,Ie1,Ie2,Ie3,Ie4,Ie5,Ie6,EnTheta')*RefAcc;

== matlab function Joint/Forward ==
  data: Theta input double; EndPos output double; L parameter double
function EndPos = fcn(Theta,L)
%#eml
gd = fwd_kin(L,Theta');
EndPos = gd(1:3,4);

== matlab function Joint/Jacobian ==
  data: Theta input double; Omega input double; EndVel output double; L parameter double
function EndVel = fcn(Theta,Omega,L)
%#eml


EndVW = spat_Jacobian(L,Theta')*Omega;
gd = fwd_kin(L,Theta');
EndW = EndVW(4:6,1);
gd_pos = gd(1:3,4);
EndVel=cross(EndW,gd_pos);

== matlab function Dynamic/Euler/N ==
  data: EnTheta input double; N output double; L_EU parameter double; Cen parameter double; Ma parameter double; Gravity parameter double
function N = fcn(EnTheta,L_EU,Cen,Ma,Gravity)
%#eml
N=zeros(6,1);
N=EulerNd(L_EU,Ma,Cen,EnTheta',Gravity);

== matlab function Dynamic/Largrange/BodyVel ==
  data: EnTheta input double; EnOmega input double; Vel output double; L parameter double; Cen parameter double
function Vel = fcn(EnTheta,EnOmega,L,Cen)
%#eml
Vel=zeros(36,1);
L=L/1000;

Vel(1:6)   = body_Jacobian_d1(L,EnTheta',Cen)*EnOmega;
Vel(7:12)  = body_Jacobian_d2(L,EnTheta',Cen)*EnOmega;
Vel(13:18) = body_Jacobian_d3(L,EnTheta',Cen)*EnOmega;
Vel(19:24) = body_Jacobian_d4(L,EnTheta',Cen)*EnOmega;
Vel(25:30) = body_Jacobian_d5(L,EnTheta',Cen)*EnOmega;
Vel(31:36) = body_Jacobian_d6(L,EnTheta',Cen)*EnOmega;
